simulink model "dds_cwg_32k_nb_half"  (R2018a)
settings: Solver=VariableStepDiscrete  StartTime=0.0  StopTime=(2^16)*20  RelTol=1e-3
undefined symbols (not defined in the file or in its folder): fft_stages, pfb_coeff_gen_calc
libraries: xbsIndex_r4 x11238, casper_library_misc x13, casper_library_delays x2, xps_library x1
(part 2 of 69)

== system dds_cwg_32k_nb_half/DDC ==
  note: DDS 18.17
  note: Mixer
  note: Filter
  note: Sync and DV will be inline here
  note: Sync and DV will be inline here
  sync : Inport
  dvalid : Inport  Port=2
  pol0_data : Inport  Port=3
  osc0 : Inport  Port=4
  pol1_data : Inport  Port=5
  osc1 : Inport  Port=6
  Assert1 : xbsIndex_r4/Assert  assert_type=on  type_source=Explicitly  gui_display_data_type=Boolean  arith_type=Boolean  n_bits=16  bin_pt=14  preci_type=Single  exp_width=8  frac_width=24  assert_rate=off  rate_source=Explicitly  period=1  output_port=on  block_type=assert
  Concat : xbsIndex_r4/Concat  num_inputs=2  dbl_ovrd=off  block_type=concat
  Concat1 : xbsIndex_r4/Concat  num_inputs=2  dbl_ovrd=off  block_type=concat
  Constant : xbsIndex_r4/Constant  const=0  gui_display_data_type=Fixed-point  arith_type=Unsigned  n_bits=1  bin_pt=0  preci_type=Single  exp_width=8  frac_width=24  explicit_period=on  period=1  equ=P=C  opselect=C  inp2=PCIN>>17  opr=+  inp1=P  carry=CIN  dbl_ovrd=off  block_type=constant
  Counter1 : xbsIndex_r4/Counter  Commented=on  cnt_type=Free Running  cnt_to=Inf  operation=Up  start_count=0  cnt_by_val=1  arith_type=Unsigned  n_bits=8  bin_pt=0  load_pin=off  rst=on  en=on  explicit_period=on  period=1  use_behavioral_HDL=off  implementation=DSP48  dbl_ovrd=off  block_type=counter
      settings: block_version=11.4
  Counter3 : xbsIndex_r4/Counter  Commented=on  cnt_type=Free Running  cnt_to=Inf  operation=Up  start_count=0  cnt_by_val=1  arith_type=Unsigned  n_bits=8  bin_pt=0  load_pin=off  rst=on  en=on  explicit_period=on  period=1  use_behavioral_HDL=off  implementation=DSP48  dbl_ovrd=off  block_type=counter
      settings: block_version=11.4
  Delay{1,9..13,15} (7 alike) : xbsIndex_r4/Delay  rst=off  infoeditControl=Selection of Reset will increase slice count due to use of real FFs and instead of SRLs  en=off  latency=1  reg_retiming=off  dbl_ovrd=off  block_type=delay
      settings: infoedit=Hardware notes: A delay line is a chain, each link of which is an SRL16 or SRL32 followed by a flip-flop.
  Delay14 : xbsIndex_r4/Delay  rst=off  infoeditControl=Selection of Reset will increase slice count due to use of real FFs and instead of SRLs  en=on  latency=2  reg_retiming=off  dbl_ovrd=off  block_type=delay
  Delay3 : xbsIndex_r4/Delay  rst=off  infoeditControl=Selection of Reset will increase slice count due to use of real FFs and instead of SRLs  en=on  latency=3  reg_retiming=off  dbl_ovrd=off  block_type=delay
  Delay4 : xbsIndex_r4/Delay  rst=off  infoeditControl=Selection of Reset will increase slice count due to use of real FFs and instead of SRLs  en=on  latency=1  reg_retiming=off  dbl_ovrd=off  block_type=delay
      settings: infoedit=Hardware notes: A delay line is a chain, each link of which is an SRL16 or SRL32 followed by a flip-flop.
  Delay5 : xbsIndex_r4/Delay  rst=off  infoeditControl=Selection of Reset will increase slice count due to use of real FFs and instead of SRLs  en=on  latency=3  reg_retiming=off  dbl_ovrd=off  block_type=delay
  Delay7 : xbsIndex_r4/Delay  rst=off  infoeditControl=Selection of Reset will increase slice count due to use of real FFs and instead of SRLs  en=on  latency=1  reg_retiming=off  dbl_ovrd=off  block_type=delay
      settings: infoedit=Hardware notes: A delay line is a chain, each link of which is an SRL16 or SRL32 followed by a flip-flop.
  Delay8 : xbsIndex_r4/Delay  rst=off  infoeditControl=Selection of Reset will increase slice count due to use of real FFs and instead of SRLs  en=on  latency=2  reg_retiming=off  dbl_ovrd=off  block_type=delay
  From16 : From  Commented=on  GotoTag=mix_80_0  TagVisibility=global
  From20 : From  Commented=on  GotoTag=cnt_rst  TagVisibility=global
      settings: CloseFcn=tagdialog Close
  From28 : From  Commented=on  GotoTag=cnt_rst  TagVisibility=global
      settings: CloseFcn=tagdialog Close
  From33 : From  Commented=on  GotoTag=dec_sync  TagVisibility=global
  From34 : From  Commented=on  GotoTag=ddc_sync
  Gateway Out{1..2,4,22..23} (5 alike) : xbsIndex_r4/Gateway Out  inherit_from_input=off  hdl_port=on  rows=1  columns=1  UseAsDAC=off  DACChannel='1'  interface=None  automatic_assignment=on  address_offset=hex2dec('00')  intf_name=''  intf_description=''  timing_constraint=None  locs_specified=off  LOCs={}  io_standard={}  block_type=gatewayout
  Gateway Out{10,12..21,24..28} (16 alike) : xbsIndex_r4/Gateway Out  Commented=on  inherit_from_input=off  hdl_port=on  rows=1  columns=1  UseAsDAC=off  DACChannel='1'  interface=None  automatic_assignment=on  address_offset=hex2dec('00')  intf_name=''  intf_description=''  timing_constraint=None  locs_specified=off  LOCs={}  io_standard={}  block_type=gatewayout
  Inverter1 : xbsIndex_r4/Inverter  en=off  latency=0  dbl_ovrd=off  block_type=inv
  Logical : xbsIndex_r4/Logical  Commented=on  logical_function=OR  inputs=2  en=off  latency=0  precision=Full  arith_type=Unsigned  n_bits=16  bin_pt=0  align_bp=on  dbl_ovrd=off  block_type=logical
  Logical3 : xbsIndex_r4/Logical  logical_function=AND  inputs=2  en=off  latency=1  precision=Full  arith_type=Unsigned  n_bits=16  bin_pt=0  align_bp=on  dbl_ovrd=off  block_type=logical
  Logical4 : xbsIndex_r4/Logical  logical_function=AND  inputs=2  en=off  latency=0  precision=Full  arith_type=Unsigned  n_bits=16  bin_pt=0  align_bp=on  dbl_ovrd=off  block_type=logical
  Register4 : xbsIndex_r4/Register  init=0  rst=off  en=on  dbl_ovrd=off  block_type=register
  Register5 : xbsIndex_r4/Register  init=0  rst=on  en=on  dbl_ovrd=off  block_type=register
  Register6 : xbsIndex_r4/Register  init=0  rst=on  en=on  dbl_ovrd=off  block_type=register
  Register7 : xbsIndex_r4/Register  init=0  rst=off  en=on  dbl_ovrd=off  block_type=register
  Terminator : Terminator
  Terminator1 : Terminator
  To Workspace1 : ToWorkspace  VariableName=mult_sync  SaveFormat=Timeseries  SampleTime=-1
  To Workspace11 : ToWorkspace  Commented=on  VariableName=mix_r0  SaveFormat=Timeseries  SampleTime=-1
  To Workspace13 : ToWorkspace  Commented=on  VariableName=mix_i0  SaveFormat=Timeseries  SampleTime=-1
  To Workspace14 : ToWorkspace  Commented=on  VariableName=mix_r1  SaveFormat=Timeseries  SampleTime=-1
  To Workspace15 : ToWorkspace  Commented=on  VariableName=mix_r2  SaveFormat=Timeseries  SampleTime=-1
  To Workspace16 : ToWorkspace  Commented=on  VariableName=mix_r3  SaveFormat=Timeseries  SampleTime=-1
  To Workspace17 : ToWorkspace  Commented=on  VariableName=mix_r4  SaveFormat=Timeseries  SampleTime=-1
  To Workspace18 : ToWorkspace  Commented=on  VariableName=mix_r5  SaveFormat=Timeseries  SampleTime=-1
  To Workspace19 : ToWorkspace  Commented=on  VariableName=mix_r6  SaveFormat=Timeseries  SampleTime=-1
  To Workspace2 : ToWorkspace  VariableName=mult_dv  SaveFormat=Timeseries  SampleTime=-1
  To Workspace20 : ToWorkspace  Commented=on  VariableName=mix_r7  SaveFormat=Timeseries  SampleTime=-1
  To Workspace21 : ToWorkspace  Commented=on  VariableName=mix_i1  SaveFormat=Timeseries  SampleTime=-1
  To Workspace22 : ToWorkspace  VariableName=ddc_pol0_re1  SaveFormat=Timeseries  SampleTime=-1
  To Workspace23 : ToWorkspace  Commented=on  VariableName=mix_i2  SaveFormat=Timeseries  SampleTime=-1
  To Workspace24 : ToWorkspace  Commented=on  VariableName=mix_i3  SaveFormat=Timeseries  SampleTime=-1
  To Workspace25 : ToWorkspace  Commented=on  VariableName=mix_i4  SaveFormat=Timeseries  SampleTime=-1
  To Workspace26 : ToWorkspace  Commented=on  VariableName=mix_i5  SaveFormat=Timeseries  SampleTime=-1
  To Workspace27 : ToWorkspace  Commented=on  VariableName=mix_i6  SaveFormat=Timeseries  SampleTime=-1
  To Workspace28 : ToWorkspace  Commented=on  VariableName=mix_i7  SaveFormat=Timeseries  SampleTime=-1
  To Workspace4 : ToWorkspace  VariableName=ddc_half_sync  SaveFormat=Timeseries  SampleTime=-1
  To Workspace5 : ToWorkspace  VariableName=ddc_pol0_im1  SaveFormat=Timeseries  SampleTime=-1
  bus_expand : Subsystem  mask(bus_expand){mode=divisions of equal size, outputNum=2, outputWidth=1, outputBinaryPt=0, outputArithmeticType=2, show_format=off, outputToWorkspace=off, variablePrefix=out, outputToModelAsWell=on}
      mask prompts: outputNum "Number of outputs:"; outputWidth "Output width:"; outputBinaryPt "Output binary point position:"; outputArithmeticType "Output arithmetic type (ufix=0, fix=1, bool=2):"; show_format "Print format string?"; outputToWorkspace "Output to workspace?"; variablePrefix "Variable name prefix:"; outputToModelAsWell "Output to model as well?"
      mask help:
      | Expands a 'bus' made using a bus_create or Xilinx
      | concat block.
      | The input will be divided into the specified number
      | of outputs with the specified arithmetic types.
      | Divisions are made from most significant bit.
      mask init: same as dds_cwg_32k_nb_half/bus_expand1
      settings: AttributesFormatString=2 outputs
      mask TypeOptions mode: divisions of equal size | divisions of arbitrary size
      mask Callback mode: bus_expand_callback();
      mask Callback outputWidth: bus_expand_callback();
      mask Callback outputToWorkspace: bus_expand_callback();
  bus_expand1 : Subsystem  mask(bus_expand){mode=divisions of equal size, outputNum=16, outputWidth=18, outputBinaryPt=17, outputArithmeticType=1, show_format=off, outputToWorkspace=off, variablePrefix=Sin, outputToModelAsWell=off}
      mask prompts: outputNum "Number of outputs:"; outputWidth "Output width:"; outputBinaryPt "Output binary point position:"; outputArithmeticType "Output arithmetic type (ufix=0, fix=1, bool=2):"; show_format "Print format string?"; outputToWorkspace "Output to workspace?"; variablePrefix "Variable name prefix:"; outputToModelAsWell "Output to model as well?"
      mask help:
      | Expands a 'bus' made using a bus_create or Xilinx
      | concat block.
      | The input will be divided into the specified number
      | of outputs with the specified arithmetic types.
      | Divisions are made from most significant bit.
      mask init: same as dds_cwg_32k_nb_half/bus_expand1
      settings: AttributesFormatString=16 outputs
      mask TypeOptions mode: divisions of equal size | divisions of arbitrary size
      mask Callback mode: bus_expand_callback();
      mask Callback outputWidth: bus_expand_callback();
      mask Callback outputToWorkspace: bus_expand_callback();
  bus_expand10 : Subsystem  mask(bus_expand){mode=divisions of equal size, outputNum=16, outputWidth=18, outputBinaryPt=17, outputArithmeticType=1, show_format=off, outputToWorkspace=off, variablePrefix=Sin, outputToModelAsWell=off}
      mask prompts: outputNum "Number of outputs:"; outputWidth "Output width:"; outputBinaryPt "Output binary point position:"; outputArithmeticType "Output arithmetic type (ufix=0, fix=1, bool=2):"; show_format "Print format string?"; outputToWorkspace "Output to workspace?"; variablePrefix "Variable name prefix:"; outputToModelAsWell "Output to model as well?"
      mask help:
      | Expands a 'bus' made using a bus_create or Xilinx
      | concat block.
      | The input will be divided into the specified number
      | of outputs with the specified arithmetic types.
      | Divisions are made from most significant bit.
      mask init: same as dds_cwg_32k_nb_half/bus_expand1
      settings: AttributesFormatString=16 outputs
      mask TypeOptions mode: divisions of equal size | divisions of arbitrary size
      mask Callback mode: bus_expand_callback();
      mask Callback outputWidth: bus_expand_callback();
      mask Callback outputToWorkspace: bus_expand_callback();
  bus_expand2 : Subsystem  mask(bus_expand){mode=divisions of equal size, outputNum=16, outputWidth=18, outputBinaryPt=17, outputArithmeticType=1, show_format=off, outputToWorkspace=off, variablePrefix=Sin, outputToModelAsWell=off}
      mask prompts: outputNum "Number of outputs:"; outputWidth "Output width:"; outputBinaryPt "Output binary point position:"; outputArithmeticType "Output arithmetic type (ufix=0, fix=1, bool=2):"; show_format "Print format string?"; outputToWorkspace "Output to workspace?"; variablePrefix "Variable name prefix:"; outputToModelAsWell "Output to model as well?"
      mask help:
      | Expands a 'bus' made using a bus_create or Xilinx
      | concat block.
      | The input will be divided into the specified number
      | of outputs with the specified arithmetic types.
      | Divisions are made from most significant bit.
      mask init: same as dds_cwg_32k_nb_half/bus_expand1
      settings: AttributesFormatString=16 outputs
      mask TypeOptions mode: divisions of equal size | divisions of arbitrary size
      mask Callback mode: bus_expand_callback();
      mask Callback outputWidth: bus_expand_callback();
      mask Callback outputToWorkspace: bus_expand_callback();
  bus_expand3 : Subsystem  mask(bus_expand){mode=divisions of equal size, outputNum=16, outputWidth=18, outputBinaryPt=17, outputArithmeticType=1, show_format=off, outputToWorkspace=off, variablePrefix=Sin, outputToModelAsWell=off}
      mask prompts: outputNum "Number of outputs:"; outputWidth "Output width:"; outputBinaryPt "Output binary point position:"; outputArithmeticType "Output arithmetic type (ufix=0, fix=1, bool=2):"; show_format "Print format string?"; outputToWorkspace "Output to workspace?"; variablePrefix "Variable name prefix:"; outputToModelAsWell "Output to model as well?"
      mask help:
      | Expands a 'bus' made using a bus_create or Xilinx
      | concat block.
      | The input will be divided into the specified number
      | of outputs with the specified arithmetic types.
      | Divisions are made from most significant bit.
      mask init: same as dds_cwg_32k_nb_half/bus_expand1
      settings: AttributesFormatString=16 outputs
      mask TypeOptions mode: divisions of equal size | divisions of arbitrary size
      mask Callback mode: bus_expand_callback();
      mask Callback outputWidth: bus_expand_callback();
      mask Callback outputToWorkspace: bus_expand_callback();
  bus_expand4 : Subsystem  mask(bus_expand){mode=divisions of equal size, outputNum=16, outputWidth=18, outputBinaryPt=17, outputArithmeticType=1, show_format=off, outputToWorkspace=off, variablePrefix=Sin, outputToModelAsWell=off}
      mask prompts: outputNum "Number of outputs:"; outputWidth "Output width:"; outputBinaryPt "Output binary point position:"; outputArithmeticType "Output arithmetic type (ufix=0, fix=1, bool=2):"; show_format "Print format string?"; outputToWorkspace "Output to workspace?"; variablePrefix "Variable name prefix:"; outputToModelAsWell "Output to model as well?"
      mask help:
      | Expands a 'bus' made using a bus_create or Xilinx
      | concat block.
      | The input will be divided into the specified number
      | of outputs with the specified arithmetic types.
      | Divisions are made from most significant bit.
      mask init: same as dds_cwg_32k_nb_half/bus_expand1
      settings: AttributesFormatString=16 outputs
      mask TypeOptions mode: divisions of equal size | divisions of arbitrary size
      mask Callback mode: bus_expand_callback();
      mask Callback outputWidth: bus_expand_callback();
      mask Callback outputToWorkspace: bus_expand_callback();
  bus_expand5 : Subsystem  mask(bus_expand){mode=divisions of equal size, outputNum=16, outputWidth=18, outputBinaryPt=17, outputArithmeticType=1, show_format=off, outputToWorkspace=off, variablePrefix=Sin, outputToModelAsWell=off}
      mask prompts: outputNum "Number of outputs:"; outputWidth "Output width:"; outputBinaryPt "Output binary point position:"; outputArithmeticType "Output arithmetic type (ufix=0, fix=1, bool=2):"; show_format "Print format string?"; outputToWorkspace "Output to workspace?"; variablePrefix "Variable name prefix:"; outputToModelAsWell "Output to model as well?"
      mask help:
      | Expands a 'bus' made using a bus_create or Xilinx
      | concat block.
      | The input will be divided into the specified number
      | of outputs with the specified arithmetic types.
      | Divisions are made from most significant bit.
      mask init: same as dds_cwg_32k_nb_half/bus_expand1
      settings: AttributesFormatString=16 outputs
      mask TypeOptions mode: divisions of equal size | divisions of arbitrary size
      mask Callback mode: bus_expand_callback();
      mask Callback outputWidth: bus_expand_callback();
      mask Callback outputToWorkspace: bus_expand_callback();
  bus_expand6 : Subsystem  mask(bus_expand){mode=divisions of equal size, outputNum=16, outputWidth=18, outputBinaryPt=17, outputArithmeticType=1, show_format=off, outputToWorkspace=off, variablePrefix=Sin, outputToModelAsWell=off}
      mask prompts: outputNum "Number of outputs:"; outputWidth "Output width:"; outputBinaryPt "Output binary point position:"; outputArithmeticType "Output arithmetic type (ufix=0, fix=1, bool=2):"; show_format "Print format string?"; outputToWorkspace "Output to workspace?"; variablePrefix "Variable name prefix:"; outputToModelAsWell "Output to model as well?"
      mask help:
      | Expands a 'bus' made using a bus_create or Xilinx
      | concat block.
      | The input will be divided into the specified number
      | of outputs with the specified arithmetic types.
      | Divisions are made from most significant bit.
      mask init: same as dds_cwg_32k_nb_half/bus_expand1
      settings: AttributesFormatString=16 outputs
      mask TypeOptions mode: divisions of equal size | divisions of arbitrary size
      mask Callback mode: bus_expand_callback();
      mask Callback outputWidth: bus_expand_callback();
      mask Callback outputToWorkspace: bus_expand_callback();
  bus_expand7 : Subsystem  AncestorBlock=casper_library_flow_control/bus_expand  mask(bus_expand){mode=divisions of equal size, outputNum=2, outputWidth=18, outputBinaryPt=17, outputArithmeticType=1, show_format=off, outputToWorkspace=off, variablePrefix=out, outputToModelAsWell=on}
      mask prompts: outputNum "Number of outputs:"; outputWidth "Output width:"; outputBinaryPt "Output binary point position:"; outputArithmeticType "Output arithmetic type (ufix=0, fix=1, bool=2):"; show_format "Print format string?"; outputToWorkspace "Output to workspace?"; variablePrefix "Variable name prefix:"; outputToModelAsWell "Output to model as well?"
      mask help:
      | Expands a 'bus' made using a bus_create or Xilinx
      | concat block.
      | The input will be divided into the specified number
      | of outputs with the specified arithmetic types.
      | Divisions are made from most significant bit.
      mask init: same as dds_cwg_32k_nb_half/bus_expand1
      settings: AttributesFormatString=2 outputs
      mask TypeOptions mode: divisions of equal size | divisions of arbitrary size
      mask Callback mode: bus_expand_callback();
      mask Callback outputWidth: bus_expand_callback();
      mask Callback outputToWorkspace: bus_expand_callback();
  bus_expand8 : Subsystem  Commented=on  mask(bus_expand){mode=divisions of equal size, outputNum=16, outputWidth=18, outputBinaryPt=17, outputArithmeticType=1, show_format=off, outputToWorkspace=off, variablePrefix=Sin, outputToModelAsWell=off}
      mask prompts: outputNum "Number of outputs:"; outputWidth "Output width:"; outputBinaryPt "Output binary point position:"; outputArithmeticType "Output arithmetic type (ufix=0, fix=1, bool=2):"; show_format "Print format string?"; outputToWorkspace "Output to workspace?"; variablePrefix "Variable name prefix:"; outputToModelAsWell "Output to model as well?"
      mask help:
      | Expands a 'bus' made using a bus_create or Xilinx
      | concat block.
      | The input will be divided into the specified number
      | of outputs with the specified arithmetic types.
      | Divisions are made from most significant bit.
      mask init: same as dds_cwg_32k_nb_half/bus_expand1
      settings: AttributesFormatString=16 outputs
      mask TypeOptions mode: divisions of equal size | divisions of arbitrary size
      mask Callback mode: bus_expand_callback();
      mask Callback outputWidth: bus_expand_callback();
      mask Callback outputToWorkspace: bus_expand_callback();
  bus_expand9 : Subsystem  mask(bus_expand){mode=divisions of equal size, outputNum=16, outputWidth=18, outputBinaryPt=17, outputArithmeticType=1, show_format=off, outputToWorkspace=off, variablePrefix=Sin, outputToModelAsWell=off}
      mask prompts: outputNum "Number of outputs:"; outputWidth "Output width:"; outputBinaryPt "Output binary point position:"; outputArithmeticType "Output arithmetic type (ufix=0, fix=1, bool=2):"; show_format "Print format string?"; outputToWorkspace "Output to workspace?"; variablePrefix "Variable name prefix:"; outputToModelAsWell "Output to model as well?"
      mask help:
      | Expands a 'bus' made using a bus_create or Xilinx
      | concat block.
      | The input will be divided into the specified number
      | of outputs with the specified arithmetic types.
      | Divisions are made from most significant bit.
      mask init: same as dds_cwg_32k_nb_half/bus_expand1
      settings: AttributesFormatString=16 outputs
      mask TypeOptions mode: divisions of equal size | divisions of arbitrary size
      mask Callback mode: bus_expand_callback();
      mask Callback outputWidth: bus_expand_callback();
      mask Callback outputToWorkspace: bus_expand_callback();
  bus_mult : Subsystem  mask(bus_mult){n_bits_a=[10,10,10,10,10,10,10,10], bin_pt_a=9, type_a=1, cmplx_a=on, n_bits_b=[18,18,18,18,18,18,18,18], bin_pt_b=17, type_b=1, cmplx_b=on, misc=on, floating_point=off, float_type=single, input_vec_a=1, input_vec_b=1, frac_width=19, exp_width=6, n_bits_out=18, bin_pt_out=17, type_out=1, quantization=1, overflow=0, mult_latency=7, add_latency=7, conv_latency=7, max_fanout=1, fan_latency=3, multiplier_implementation=embedded multiplier core, pipeline_cmult_en=off, pipeline_latency=0}
      mask prompts: n_bits_a "a input bit widths"; bin_pt_a "a input binary points"; type_a "a input type (Unsigned=0, Signed=1)"; cmplx_a "a input complex"; n_bits_b "b input bit widths"; bin_pt_b "b input binary points"; type_b "b input type (Unsigned=0, Signed=1)"; cmplx_b "b input complex"; misc "misc support"; floating_point "floating point"; float_type "float type"; input_vec_a "a input vector in bus"; input_vec_b "b input vector in bus"; frac_width "fraction width"; exp_width "exponent width"; n_bits_out "output bit widths"; bin_pt_out "output binary points"; type_out "output type (Unsigned=0, Signed=1)"; quantization "quantization strategy (Truncate=0, Round  (unbiased: +/- Inf)=1)"; overflow "overflow strategy (Wrap=0, Saturate=1, Flag as error=2)"; mult_latency "multiplier latency"; add_latency "adder latency"; conv_latency "convert latency"; max_fanout "limit fanout to ?"; fan_latency "fanout register latency"; multiplier_implementation "multiplier implementation"; pipeline_cmult_en "pipeline complex mult"; pipeline_latency "pipeline latency"
      mask help: Multiply components of two busses
      mask init:
      | bus_mult_init(gcb, ...
      |     'n_bits_a', n_bits_a, ...
      |     'bin_pt_a', bin_pt_a, ...
      |     'type_a', type_a, ...
      |     'cmplx_a', cmplx_a, ...
      |     'n_bits_b', n_bits_b, ...
      |     'bin_pt_b', bin_pt_b, ...
      |     'type_b', type_b, ...
      |     'cmplx_b', cmplx_b, ...
      |     'n_bits_out', n_bits_out, ...
      |     'bin_pt_out', bin_pt_out, ...
      |     'type_out', type_out, ...
      |     'floating_point', floating_point, ...
      |     'float_type', float_type, ...
      |     'exp_width', exp_width, ...
      |     'input_vec_a', input_vec_a, ...
      |     'input_vec_b', input_vec_b, ...
      |     'frac_width', frac_width, ...         
      |     'quantization', quantization, ...
      |     'overflow', overflow, ...
      |     'mult_latency', mult_latency, ...
      |     'add_latency', add_latency, ...
      |     'conv_latency', conv_latency, ...
      |     'max_fanout', max_fanout, ...
      |     'pipeline_cmult_en', pipeline_cmult_en, ...
      |     'pipeline_latency', pipeline_latency, ...
      |     'fan_latency', fan_latency, ...
      |     'multiplier_implementation', multiplier_implementation, ...
      |     'misc', misc);
      mask Callback floating_point:
      | onoff = get_param(gcb, 'floating_point');
      | if strcmp(onoff,'on')
      |     enable_fixpt = 'off'
      |     set_param_state(gcb, 'float_type', 'on')
      | 
      |     set_param_state(gcb, 'input_vec_a', 'on')
      |     set_param_state(gcb, 'input_vec_b', 'on')
      | 
      |     f_type = get_param(gcb, 'float_type')
      |     if strcmp(f_type,'custom')
      |         set_param_state(gcb, 'exp_width', 'on')
      |         set_param_state(gcb, 'frac_width', 'on')
      |     else
      |         set_param_state(gcb, 'exp_width', 'off')
      |         set_param_state(gcb, 'frac_width', 'off')
      |     end
      | 
      | else
      |     enable_fixpt = 'on'
      |     set_param_state(gcb, 'float_type', 'off')
      |     set_param_state(gcb, 'exp_width', 'off')
      |     set_param_state(gcb, 'frac_width', 'off')
      |     set_param_state(gcb, 'input_vec_a', 'off')
      |     set_param_state(gcb, 'input_vec_b', 'off')
      | end
      | 
      | set_param_state(gcb, 'n_bits_a', enable_fixpt)
      | set_param_state(gcb, 'bin_pt_a', enable_fixpt)
      | set_param_state(gcb, 'type_a', enable_fixpt)
      | set_param_state(gcb, 'n_bits_b', enable_fixpt)
      | set_param_state(gcb, 'bin_pt_b', enable_fixpt)
      | set_param_state(gcb, 'type_b', enable_fixpt)
      | 
      | set_param_state(gcb, 'n_bits_out', enable_fixpt)
      | set_param_state(gcb, 'bin_pt_out', enable_fixpt)
      | set_param_state(gcb, 'type_out', enable_fixpt)
      | set_param_state(gcb, 'quantization', enable_fixpt)
      | set_param_state(gcb, 'overflow', enable_fixpt)
      mask TypeOptions float_type: single | custom
      mask Callback float_type:
      | f_type = get_param(gcb, 'float_type')
      | if strcmp(f_type,'custom')
      |     set_param_state(gcb, 'exp_width', 'on')
      |     set_param_state(gcb, 'frac_width', 'on')
      | else
      |     set_param_state(gcb, 'exp_width', 'off')
      |     set_param_state(gcb, 'frac_width', 'off')
      | end
      mask TypeOptions multiplier_implementation: behavioral HDL | standard core | embedded multiplier core
      mask Callback pipeline_cmult_en:
      | pipeline_en = get_param(gcb, 'pipeline_cmult_en');
      | if strcmp(pipeline_en,'on')
      | 
      |     set_param_state(gcb, 'pipeline_latency', 'on')
      | else
      |     set_param_state(gcb, 'pipeline_latency', 'off')
      | end
  bus_mult1 : Subsystem  mask(bus_mult){n_bits_a=[10,10,10,10,10,10,10,10], bin_pt_a=9, type_a=1, cmplx_a=on, n_bits_b=[18,18,18,18,18,18,18,18], bin_pt_b=17, type_b=1, cmplx_b=on, misc=off, floating_point=off, float_type=single, input_vec_a=1, input_vec_b=1, frac_width=19, exp_width=6, n_bits_out=18, bin_pt_out=17, type_out=1, quantization=1, overflow=0, mult_latency=7, add_latency=7, conv_latency=7, max_fanout=1, fan_latency=3, multiplier_implementation=embedded multiplier core, pipeline_cmult_en=off, pipeline_latency=0}
      mask prompts: n_bits_a "a input bit widths"; bin_pt_a "a input binary points"; type_a "a input type (Unsigned=0, Signed=1)"; cmplx_a "a input complex"; n_bits_b "b input bit widths"; bin_pt_b "b input binary points"; type_b "b input type (Unsigned=0, Signed=1)"; cmplx_b "b input complex"; misc "misc support"; floating_point "floating point"; float_type "float type"; input_vec_a "a input vector in bus"; input_vec_b "b input vector in bus"; frac_width "fraction width"; exp_width "exponent width"; n_bits_out "output bit widths"; bin_pt_out "output binary points"; type_out "output type (Unsigned=0, Signed=1)"; quantization "quantization strategy (Truncate=0, Round  (unbiased: +/- Inf)=1)"; overflow "overflow strategy (Wrap=0, Saturate=1, Flag as error=2)"; mult_latency "multiplier latency"; add_latency "adder latency"; conv_latency "convert latency"; max_fanout "limit fanout to ?"; fan_latency "fanout register latency"; multiplier_implementation "multiplier implementation"; pipeline_cmult_en "pipeline complex mult"; pipeline_latency "pipeline latency"
      mask help: Multiply components of two busses
      mask init: same as dds_cwg_32k_nb_half/DDC/bus_mult
      mask Callback floating_point:
      | onoff = get_param(gcb, 'floating_point');
      | if strcmp(onoff,'on')
      |     enable_fixpt = 'off'
      |     set_param_state(gcb, 'float_type', 'on')
      | 
      |     set_param_state(gcb, 'input_vec_a', 'on')
      |     set_param_state(gcb, 'input_vec_b', 'on')
      | 
      |     f_type = get_param(gcb, 'float_type')
      |     if strcmp(f_type,'custom')
      |         set_param_state(gcb, 'exp_width', 'on')
      |         set_param_state(gcb, 'frac_width', 'on')
      |     else
      |         set_param_state(gcb, 'exp_width', 'off')
      |         set_param_state(gcb, 'frac_width', 'off')
      |     end
      | 
      | else
      |     enable_fixpt = 'on'
      |     set_param_state(gcb, 'float_type', 'off')
      |     set_param_state(gcb, 'exp_width', 'off')
      |     set_param_state(gcb, 'frac_width', 'off')
      |     set_param_state(gcb, 'input_vec_a', 'off')
      |     set_param_state(gcb, 'input_vec_b', 'off')
      | end
      | 
      | set_param_state(gcb, 'n_bits_a', enable_fixpt)
      | set_param_state(gcb, 'bin_pt_a', enable_fixpt)
      | set_param_state(gcb, 'type_a', enable_fixpt)
      | set_param_state(gcb, 'n_bits_b', enable_fixpt)
      | set_param_state(gcb, 'bin_pt_b', enable_fixpt)
      | set_param_state(gcb, 'type_b', enable_fixpt)
      | 
      | set_param_state(gcb, 'n_bits_out', enable_fixpt)
      | set_param_state(gcb, 'bin_pt_out', enable_fixpt)
      | set_param_state(gcb, 'type_out', enable_fixpt)
      | set_param_state(gcb, 'quantization', enable_fixpt)
      | set_param_state(gcb, 'overflow', enable_fixpt)
      mask TypeOptions float_type: single | custom
      mask Callback float_type:
      | f_type = get_param(gcb, 'float_type')
      | if strcmp(f_type,'custom')
      |     set_param_state(gcb, 'exp_width', 'on')
      |     set_param_state(gcb, 'frac_width', 'on')
      | else
      |     set_param_state(gcb, 'exp_width', 'off')
      |     set_param_state(gcb, 'frac_width', 'off')
      | end
      mask TypeOptions multiplier_implementation: behavioral HDL | standard core | embedded multiplier core
      mask Callback pipeline_cmult_en:
      | pipeline_en = get_param(gcb, 'pipeline_cmult_en');
      | if strcmp(pipeline_en,'on')
      | 
      |     set_param_state(gcb, 'pipeline_latency', 'on')
      | else
      |     set_param_state(gcb, 'pipeline_latency', 'off')
      | end
  convert_of : Subsystem  Commented=on  AncestorBlock=casper_library_misc/convert_of  mask(convert_of){bit_width_i=44, binary_point_i=34, bit_width_o=18, binary_point_o=17, latency=2, overflow=Saturate, quantization=Round  (unbiased: +/- Inf)}
      mask prompts: bit_width_i "Bit Width In"; binary_point_i "Binary Point In"; bit_width_o "Bit Width Out"; binary_point_o "Binary Point Out"; overflow "Overflow Behaviour"; quantization "Quantization Behaviour"
      mask help:
      | Converts from one 2's complement bit-width
      | and/or binary point position to another.
      | Includes underflow/overflow indicator.
      mask init:
      | convert_of_init(gcb, ...
      |     'bit_width_i', bit_width_i, ...
      |     'binary_point_i', binary_point_i, ...
      |     'bit_width_o', bit_width_o, ...
      |     'binary_point_o', binary_point_o, ...
      |     'latency', latency, ...
      |     'overflow', overflow, ...
      |     'quantization', quantization);
      settings: AttributesFormatString=[44,34]->[18,17]
      mask TypeOptions overflow: Wrap | Saturate | Error
      mask TypeOptions quantization: Truncate | Round  (unbiased: +/- Inf) | Round  (unbiased: even values)
  convert_of1 : Subsystem  Commented=on  AncestorBlock=casper_library_misc/convert_of  mask(convert_of){bit_width_i=44, binary_point_i=34, bit_width_o=18, binary_point_o=17, latency=2, overflow=Saturate, quantization=Round  (unbiased: +/- Inf)}
      mask prompts: bit_width_i "Bit Width In"; binary_point_i "Binary Point In"; bit_width_o "Bit Width Out"; binary_point_o "Binary Point Out"; overflow "Overflow Behaviour"; quantization "Quantization Behaviour"
      mask help:
      | Converts from one 2's complement bit-width
      | and/or binary point position to another.
      | Includes underflow/overflow indicator.
      mask init: same as dds_cwg_32k_nb_half/DDC/convert_of
      settings: AttributesFormatString=[44,34]->[18,17]
      mask TypeOptions overflow: Wrap | Saturate | Error
      mask TypeOptions quantization: Truncate | Round  (unbiased: +/- Inf) | Round  (unbiased: even values)
  ddc_in_sync_cnt : Subsystem  Tag=xps:sw_reg  Commented=on  AncestorBlock=xps_library/Memory/software_register  mask(swreg){io_dir=To Processor, io_delay=0, init_val=0, sample_period=1, names=reg, bitwidths=8, bin_pts=0, arith_types=0, sim_port=off, show_format=on}
      mask prompts: io_dir "I/O direction"; io_delay "I/O delay"; init_val "Initial Value"; sample_period "Sample period"; names "Bitfield names [msb...lsb]"; bitwidths "Bitfield widths"; bin_pts "Bitfield binary pts"; arith_types "Bitfield types, ufix=0, fix=1, bool=2"; sim_port "Provide sim input/output?"; show_format "Print format string?"
      mask help: A 32-bit software-accessible register. Can be divided into bitfields of varying widths and types using the fields in the block mask.
      mask init:
      | swreg_init(gcb)
      settings: AttributesFormatString=1output:uf8.0 = 8 bits
      mask TypeOptions io_dir: To Processor | From Processor
      mask Callback io_dir:
      | mask_enables = get_param(gcb, 'MaskEnables');
      | mask_names = get_param(gcb, 'MaskNames');
      | if strcmp(get_param(gcb, 'io_dir'), 'To Processor'),
      |     mask_enables{ismember(mask_names, 'sample_period')} = 'off';
      | else
      |     mask_enables{ismember(mask_names, 'sample_period')} = 'on';
      | end
      | set_param(gcb, 'MaskEnables', mask_enables);
      mask DialogControl ParameterTabVar0 Prompt: Setup
  ddc_out_sync_cnt : Subsystem  Tag=xps:sw_reg  Commented=on  AncestorBlock=xps_library/Memory/software_register  mask(swreg){io_dir=To Processor, io_delay=0, init_val=0, sample_period=1, names=reg, bitwidths=8, bin_pts=0, arith_types=0, sim_port=off, show_format=on}
      mask prompts: io_dir "I/O direction"; io_delay "I/O delay"; init_val "Initial Value"; sample_period "Sample period"; names "Bitfield names [msb...lsb]"; bitwidths "Bitfield widths"; bin_pts "Bitfield binary pts"; arith_types "Bitfield types, ufix=0, fix=1, bool=2"; sim_port "Provide sim input/output?"; show_format "Print format string?"
      mask help: A 32-bit software-accessible register. Can be divided into bitfields of varying widths and types using the fields in the block mask.
      mask init:
      | swreg_init(gcb)
      settings: AttributesFormatString=1output:uf8.0 = 8 bits
      mask TypeOptions io_dir: To Processor | From Processor
      mask Callback io_dir:
      | mask_enables = get_param(gcb, 'MaskEnables');
      | mask_names = get_param(gcb, 'MaskNames');
      | if strcmp(get_param(gcb, 'io_dir'), 'To Processor'),
      |     mask_enables{ismember(mask_names, 'sample_period')} = 'off';
      | else
      |     mask_enables{ismember(mask_names, 'sample_period')} = 'on';
      | end
      | set_param(gcb, 'MaskEnables', mask_enables);
      mask DialogControl ParameterTabVar0 Prompt: Setup
  dec_fir_async1 : Subsystem  Tag=casper:dec_fir_async  AncestorBlock=casper_library_downconverter/dec_fir_async  mask(dec_fir_async){n_inputs=32, coeff=[-0.000339,-0.000234,-0.000312,-0.000402,-0.000507,-0.000626,-0.000760,-0.000909,-0.001071,-0.001247,-0.001436,-0.001634,-0.001841,-0.002054,-0.002269,-0.002483,-0.002692,-0.002892,-0.003077,-0.003243,-0.003383,-0.003491,-0.003562,-0.003589,-0.003566,-0.003487,-0.003345,-0.003135,-0.002850,-0.002487,-0.002040,-0.001506,-0.000881,-0.000163,0.000649,0.001555,0.002555,0.003646,0.004826,0.006089,0.007432,0.008847,0.010325,0.011860,0.013440,0.015055,0.016693,0.018341,0.019988,0.021620,0.023223,0.024783,0.026286,0.027720,0.029072,0.030327,0.031476,0.032507,0.033410,0.034177,0.034799,0.035272,0.035589,0.035749,0.035749,0.035589,0.035272,0.034799,0.034177,0.033410,0.032507,0.031476,0.030327,0.029072,0.027720,0.026286,0.024783,0.023223,0.021620,0.019988,0.018341,0.016693,0.015055,0.013440,0.011860,0.010325,0.008847,0.007432,0.006089,0.004826,0.003646,0.002555,0.001555,0.000649,-0.000163,-0.000881,-0.001506,-0.002040,-0.002487,-0.002850,-0.003135,-0.003345,-0.003487,-0.003566,-0.003589,-0.003562,-0.003491,-0.003383,-0.003243,-0.003077,-0.002892,-0.002692,-0.002483,-0.002269,-0.002054,-0.001841,-0.001634,-0.001436,-0.001247,-0.001071,-0.000909,-0.000760,-0.000626,-0.000507,-0.000402,-0.000312,-0.000234,-0.000339], output_width=18, output_bp=17, quantization=Round  (unbiased: +/- Inf), add_latency=7, mult_latency=7, conv_latency=7, coeff_bit_width=18, coeff_bin_pt=17, lshift=1, absorb_adders=on, adder_imp=DSP48, async=on, bus_input=off, input_width=0, input_bp=0, input_type=Signed}
      mask prompts: n_inputs "Number of Parallel Streams"; coeff "Coefficients"; output_width "Output bitwidth"; output_bp "Output binary point"; quantization "Quantization Behavior"; add_latency "Add Latency"; mult_latency "Mult Latency"; conv_latency "Convert latency"; coeff_bit_width "Coefficient bitwidth"; coeff_bin_pt "Coefficient binary point"; lshift "Post adder-tree shift"; absorb_adders "Absorb adders into DSP slices"; adder_imp "Adder implementation"; async "Asynchronous ops"; bus_input "Bus input"; input_width "Input bitwidth"; input_bp "Input binary point"; input_type "Input datatype"
      mask help: FIR filter which can handle multiple time samples in parallel and decimates down to 1 time sample. If coefficients are symmetric, will automatically fold before multiplying.
      mask init:
      | dec_fir_async_init(gcb);
      settings: AttributesFormatString=|
      | 128 taps
      | 18_17 r/i
      mask TypeOptions quantization: Truncate | Round  (unbiased: +/- Inf) | Round  (unbiased: Even Values)
      mask TypeOptions adder_imp: Behavioral | Fabric | DSP48
      mask Callback bus_input:
      | onoff = get_param(gcb, 'bus_input');
      | set_param_state(gcb, 'input_width', onoff)
      | set_param_state(gcb, 'input_bp', onoff)
      | set_param_state(gcb, 'input_type', onoff)
      mask TypeOptions input_type: Signed | Unsigned
  dec_fir_async2 : Subsystem  Tag=casper:dec_fir_async  AncestorBlock=casper_library_downconverter/dec_fir_async  mask(dec_fir_async){n_inputs=32, coeff=[-0.000339,-0.000234,-0.000312,-0.000402,-0.000507,-0.000626,-0.000760,-0.000909,-0.001071,-0.001247,-0.001436,-0.001634,-0.001841,-0.002054,-0.002269,-0.002483,-0.002692,-0.002892,-0.003077,-0.003243,-0.003383,-0.003491,-0.003562,-0.003589,-0.003566,-0.003487,-0.003345,-0.003135,-0.002850,-0.002487,-0.002040,-0.001506,-0.000881,-0.000163,0.000649,0.001555,0.002555,0.003646,0.004826,0.006089,0.007432,0.008847,0.010325,0.011860,0.013440,0.015055,0.016693,0.018341,0.019988,0.021620,0.023223,0.024783,0.026286,0.027720,0.029072,0.030327,0.031476,0.032507,0.033410,0.034177,0.034799,0.035272,0.035589,0.035749,0.035749,0.035589,0.035272,0.034799,0.034177,0.033410,0.032507,0.031476,0.030327,0.029072,0.027720,0.026286,0.024783,0.023223,0.021620,0.019988,0.018341,0.016693,0.015055,0.013440,0.011860,0.010325,0.008847,0.007432,0.006089,0.004826,0.003646,0.002555,0.001555,0.000649,-0.000163,-0.000881,-0.001506,-0.002040,-0.002487,-0.002850,-0.003135,-0.003345,-0.003487,-0.003566,-0.003589,-0.003562,-0.003491,-0.003383,-0.003243,-0.003077,-0.002892,-0.002692,-0.002483,-0.002269,-0.002054,-0.001841,-0.001634,-0.001436,-0.001247,-0.001071,-0.000909,-0.000760,-0.000626,-0.000507,-0.000402,-0.000312,-0.000234,-0.000339], output_width=18, output_bp=17, quantization=Round  (unbiased: +/- Inf), add_latency=7, mult_latency=7, conv_latency=7, coeff_bit_width=18, coeff_bin_pt=17, lshift=1, absorb_adders=on, adder_imp=DSP48, async=on, bus_input=off, input_width=0, input_bp=0, input_type=Signed}
      mask prompts: n_inputs "Number of Parallel Streams"; coeff "Coefficients"; output_width "Output bitwidth"; output_bp "Output binary point"; quantization "Quantization Behavior"; add_latency "Add Latency"; mult_latency "Mult Latency"; conv_latency "Convert latency"; coeff_bit_width "Coefficient bitwidth"; coeff_bin_pt "Coefficient binary point"; lshift "Post adder-tree shift"; absorb_adders "Absorb adders into DSP slices"; adder_imp "Adder implementation"; async "Asynchronous ops"; bus_input "Bus input"; input_width "Input bitwidth"; input_bp "Input binary point"; input_type "Input datatype"
      mask help: FIR filter which can handle multiple time samples in parallel and decimates down to 1 time sample. If coefficients are symmetric, will automatically fold before multiplying.
      mask init:
      | dec_fir_async_init(gcb);
      settings: AttributesFormatString=|
      | 128 taps
      | 18_17 r/i
      mask TypeOptions quantization: Truncate | Round  (unbiased: +/- Inf) | Round  (unbiased: Even Values)
      mask TypeOptions adder_imp: Behavioral | Fabric | DSP48
      mask Callback bus_input:
      | onoff = get_param(gcb, 'bus_input');
      | set_param_state(gcb, 'input_width', onoff)
      | set_param_state(gcb, 'input_bp', onoff)
      | set_param_state(gcb, 'input_type', onoff)
      mask TypeOptions input_type: Signed | Unsigned
  edge_detect2 : Subsystem  AncestorBlock=casper_library_misc/edge_detect  mask(edge_detect){edge=Rising, polarity=Active High, x_in=[0 0.08 0.08 0.16 0.16 0.24 0.24 0.32 0.32 0.4], y_in=[-1 -1  1  1  1  1  1  1  1  1], x_out=[0.6 0.68 0.68 0.76 0.76 0.84 0.84 0.92 0.92 1], y_out=[-1 -1  1  1 -1 -1 -1 -1 -1 -1]}
      mask prompts: edge "Edge Type"; polarity "Output Polarity"; x_in "Input X Positions"; y_in "Input Y Positions"; x_out "Output X Positions"; y_out "Output Y Positions"
      mask help: Output is active for one-cycle after each edge of the specified type (i.e. rising, falling or both).
      mask init: same as dds_cwg_32k_nb_half/edge_detect1
      settings: AttributesFormatString=|
      | rising edges
      | active high
      mask Help: Output is active for one-cycle after each edge of the specified type (i.e. rising, falling, or both).  Latency is zero.
      mask TypeOptions edge: Rising | Falling | Both
      mask TypeOptions polarity: Active High | Active Low
      mask Display:
      | plot(x_in_num,0.5+y_in_num*0.2);
      | plot(x_out_num,0.5+y_out_num*0.2);
  pipeline21 : Subsystem  Commented=on  AncestorBlock=casper_library_delays/pipeline  mask(pipeline){latency=2}
      mask help:
      | An explicitly laid-out delay line to avoid mapping to SRL16s
      | for use in pipelining to help achieve timing closure.
      mask init:
      | pipeline_init(gcb,'latency',latency);
      settings: AttributesFormatString=Latency = %<latency>
      mask Display:
      | port_label('input', 1, 'd');
      | port_label('output', 1, 'q');
      | disp(['Z^-', num2str(latency)]);
  pipeline22 : Subsystem  Commented=on  AncestorBlock=casper_library_delays/pipeline  mask(pipeline){latency=2}
      mask help:
      | An explicitly laid-out delay line to avoid mapping to SRL16s
      | for use in pipelining to help achieve timing closure.
      mask init:
      | pipeline_init(gcb,'latency',latency);
      settings: AttributesFormatString=Latency = %<latency>
      mask Display:
      | port_label('input', 1, 'd');
      | port_label('output', 1, 'q');
      | disp(['Z^-', num2str(latency)]);
  pipeline39 : Subsystem  Commented=on  AncestorBlock=casper_library_delays/pipeline  mask(pipeline){latency=2}
      mask help:
      | An explicitly laid-out delay line to avoid mapping to SRL16s
      | for use in pipelining to help achieve timing closure.
      mask init:
      | pipeline_init(gcb,'latency',latency);
      settings: AttributesFormatString=Latency = %<latency>
      mask Display:
      | port_label('input', 1, 'd');
      | port_label('output', 1, 'q');
      | disp(['Z^-', num2str(latency)]);
  pipeline40 : Subsystem  Commented=on  AncestorBlock=casper_library_delays/pipeline  mask(pipeline){latency=2}
      mask help:
      | An explicitly laid-out delay line to avoid mapping to SRL16s
      | for use in pipelining to help achieve timing closure.
      mask init:
      | pipeline_init(gcb,'latency',latency);
      settings: AttributesFormatString=Latency = %<latency>
      mask Display:
      | port_label('input', 1, 'd');
      | port_label('output', 1, 'q');
      | disp(['Z^-', num2str(latency)]);
  ri_to_c1 : casper_library_misc/ri_to_c  Commented=on
      settings: SourceProductName=CASPER DSP Blockset
  ddc_sync : Outport
  ddc_pol0 : Outport  Port=2
  ddc_pol1 : Outport  Port=3
  ddc_dv : Outport  Port=4
  ddc_of : Outport  Port=5
  tag scope: dec_d80_0=global, dec_d80_1=global, dec_dv=global, dec_sync=global, mix_80_0=global, mix_dvalid=global, mix_sync=global
  wires:
  Concat/1 -> bus_mult/3(misci)
  bus_mult/2(misco) -> bus_expand/1(bus_in)
  [ddc_sync] -> ddc_sync/1
  [ddc_pol0] -> ddc_pol0/1
  [ddc_pol1] -> ddc_pol1/1
  pol1_data/1 -> bus_mult1/1(a)
  osc1/1 -> bus_mult1/2(b)
  From20/1 -> pipeline22/1(d)
  Counter1/1 -> ddc_out_sync_cnt/1(out_reg)
  pipeline21/1(q) -> Counter1/2
  pipeline22/1(q) -> Counter1/1
  From34/1 -> pipeline21/1(d)
  [ddc_dvalid] -> ddc_dv/1
  From28/1 -> pipeline40/1(d)
  Counter3/1 -> ddc_in_sync_cnt/1(out_reg)
  pipeline39/1(q) -> Counter3/2
  pipeline40/1(q) -> Counter3/1
  From33/1 -> pipeline39/1(d)
  [ddc_of_pol0] -> Concat1/1
  [ddc_of_pol1] -> Concat1/2
  Concat1/1 -> ddc_of/1
  Constant/1 -> [ddc_of_pol1], [ddc_of_pol0]
  convert_of1/1(dout) -> ri_to_c1/2
  convert_of/1(dout) -> ri_to_c1/1
  convert_of/2(of) -> Logical/1
  convert_of1/2(of) -> Logical/2
  sync/1 -> Concat/1
  dvalid/1 -> Concat/2
  osc0/1 -> bus_mult/2(b)
  pol0_data/1 -> bus_mult/1(a)
  bus_expand/1(msb_out2) -> Gateway Out1/1, [mix_sync]
  Gateway Out1/1 -> To Workspace1/1
  Gateway Out2/1 -> To Workspace2/1
  bus_expand/2(lsb_out1) -> Gateway Out2/1, [mix_dvalid]
  bus_mult1/1(a*b) -> [mix_80_1]
  bus_mult/1(a*b) -> [mix_80_0]
  [dec_d80_0] -> Delay5/1, Delay8/1, Delay7/1, bus_expand4/1(bus_in)
  [dec_dv] -> dec_fir_async1/2(dv_in)
  [dec_sync] -> dec_fir_async1/1(sync_in)
  bus_expand1/1(msb_out16) -> dec_fir_async1/3(real1)
  bus_expand1/2(out15) -> dec_fir_async1/4(imag1)
  bus_expand1/3(out14) -> dec_fir_async1/5(real2)
  bus_expand1/4(out13) -> dec_fir_async1/6(imag2)
  bus_expand1/5(out12) -> dec_fir_async1/7(real3)
  bus_expand1/6(out11) -> dec_fir_async1/8(imag3)
  bus_expand1/7(out10) -> dec_fir_async1/9(real4)
  bus_expand1/8(out9) -> dec_fir_async1/10(imag4)
  bus_expand1/9(out8) -> dec_fir_async1/11(real5)
  bus_expand1/10(out7) -> dec_fir_async1/12(imag5)
  bus_expand1/11(out6) -> dec_fir_async1/13(real6)
  bus_expand1/12(out5) -> dec_fir_async1/14(imag6)
  bus_expand1/13(out4) -> dec_fir_async1/15(real7)
  bus_expand1/14(out3) -> dec_fir_async1/16(imag7)
  bus_expand1/15(out2) -> dec_fir_async1/17(real8)
  bus_expand1/16(lsb_out1) -> dec_fir_async1/18(imag8)
  bus_expand2/1(msb_out16) -> dec_fir_async1/19(real9)
  bus_expand2/2(out15) -> dec_fir_async1/20(imag9)
  bus_expand2/3(out14) -> dec_fir_async1/21(real10)
  bus_expand2/4(out13) -> dec_fir_async1/22(imag10)
  bus_expand2/5(out12) -> dec_fir_async1/23(real11)
  bus_expand2/6(out11) -> dec_fir_async1/24(imag11)
  bus_expand2/7(out10) -> dec_fir_async1/25(real12)
  bus_expand2/8(out9) -> dec_fir_async1/26(imag12)
  bus_expand2/9(out8) -> dec_fir_async1/27(real13)
  bus_expand2/10(out7) -> dec_fir_async1/28(imag13)
  bus_expand2/11(out6) -> dec_fir_async1/29(real14)
  bus_expand2/12(out5) -> dec_fir_async1/30(imag14)
  bus_expand2/13(out4) -> dec_fir_async1/31(real15)
  bus_expand2/14(out3) -> dec_fir_async1/32(imag15)
  bus_expand2/15(out2) -> dec_fir_async1/33(real16)
  bus_expand2/16(lsb_out1) -> dec_fir_async1/34(imag16)
  Delay5/1 -> bus_expand1/1(bus_in)
  bus_expand3/1(msb_out16) -> dec_fir_async1/35(real17)
  bus_expand3/2(out15) -> dec_fir_async1/36(imag17)
  bus_expand3/3(out14) -> dec_fir_async1/37(real18)
  bus_expand3/4(out13) -> dec_fir_async1/38(imag18)
  bus_expand3/5(out12) -> dec_fir_async1/39(real19)
  bus_expand3/6(out11) -> dec_fir_async1/40(imag19)
  bus_expand3/7(out10) -> dec_fir_async1/41(real20)
  bus_expand3/9(out8) -> dec_fir_async1/43(real21)
  bus_expand3/8(out9) -> dec_fir_async1/42(imag20)
  bus_expand3/10(out7) -> dec_fir_async1/44(imag21)
  bus_expand3/11(out6) -> dec_fir_async1/45(real22)
  bus_expand3/12(out5) -> dec_fir_async1/46(imag22)
  bus_expand3/13(out4) -> dec_fir_async1/47(real23)
  bus_expand3/14(out3) -> dec_fir_async1/48(imag23)
  bus_expand3/15(out2) -> dec_fir_async1/49(real24)
  bus_expand3/16(lsb_out1) -> dec_fir_async1/50(imag24)
  bus_expand4/1(msb_out16) -> dec_fir_async1/51(real25)
  bus_expand4/2(out15) -> dec_fir_async1/52(imag25)
  bus_expand4/3(out14) -> dec_fir_async1/53(real26)
  bus_expand4/4(out13) -> dec_fir_async1/54(imag26)
  bus_expand4/5(out12) -> dec_fir_async1/55(real27)
  bus_expand4/6(out11) -> dec_fir_async1/56(imag27)
  bus_expand4/7(out10) -> dec_fir_async1/57(real28)
  bus_expand4/8(out9) -> dec_fir_async1/58(imag28)
  bus_expand4/9(out8) -> dec_fir_async1/59(real29)
  bus_expand4/10(out7) -> dec_fir_async1/60(imag29)
  bus_expand4/11(out6) -> dec_fir_async1/61(real30)
  bus_expand4/13(out4) -> dec_fir_async1/63(real31)
  bus_expand4/12(out5) -> dec_fir_async1/62(imag30)
  bus_expand4/14(out3) -> dec_fir_async1/64(imag31)
  bus_expand4/15(out2) -> dec_fir_async1/65(real32)
  bus_expand4/16(lsb_out1) -> dec_fir_async1/66(imag32)
  Delay7/1 -> bus_expand3/1(bus_in)
  [mix_dvalid] -> Delay5/2, Delay8/2, Delay7/2
  Delay8/1 -> bus_expand2/1(bus_in)
  dec_fir_async1/2(dout) -> Delay10/1
  dec_fir_async1/3(dv_out) -> Delay9/1
  Delay9/1 -> [ddc_dvalid]
  Gateway Out4/1 -> To Workspace4/1
  bus_expand7/1(msb_out2) -> Gateway Out22/1
  bus_expand7/2(lsb_out1) -> Gateway Out23/1
  Gateway Out22/1 -> To Workspace22/1
  Gateway Out23/1 -> To Workspace5/1
  [mix_80_1] -> Register7/1
  [mix_80_0] -> Register4/1
  [mix_dvalid] -> Register5/3, Logical3/2, Register4/2, Register7/2
  Logical4/1 -> Delay12/1, Register6/2
  Register6/1 -> Logical4/1
  [mix_sync] -> Register6/1, Register6/3, Register5/2
  Assert1/1 -> Register5/1
  Inverter1/1 -> Assert1/1
  Register5/1 -> Delay13/1
  Delay13/1 -> Logical3/1, Inverter1/1
  Delay12/1 -> [dec_sync]
  Delay11/1 -> [dec_dv]
  Register4/1 -> [dec_d80_0]
  Register7/1 -> [dec_d80_1]
  Logical3/1 -> edge_detect2/1(in), Logical4/2
  edge_detect2/1(out) -> Delay11/1
  From16/1 -> bus_expand8/1(bus_in)
  Gateway Out10/1 -> To Workspace11/1
  bus_expand8/1(msb_out16) -> Gateway Out10/1
  Gateway Out12/1 -> To Workspace13/1
  bus_expand8/2(out15) -> Gateway Out12/1
  Gateway Out13/1 -> To Workspace14/1
  bus_expand8/3(out14) -> Gateway Out13/1
  Gateway Out14/1 -> To Workspace21/1
  bus_expand8/4(out13) -> Gateway Out14/1
  Gateway Out18/1 -> To Workspace24/1
  Gateway Out17/1 -> To Workspace16/1
  Gateway Out16/1 -> To Workspace23/1
  Gateway Out15/1 -> To Workspace15/1
  bus_expand8/5(out12) -> Gateway Out15/1
  bus_expand8/6(out11) -> Gateway Out16/1
  bus_expand8/7(out10) -> Gateway Out17/1
  bus_expand8/8(out9) -> Gateway Out18/1
  Gateway Out25/1 -> To Workspace19/1
  Gateway Out26/1 -> To Workspace27/1
  Gateway Out27/1 -> To Workspace20/1
  Gateway Out28/1 -> To Workspace28/1
  Gateway Out24/1 -> To Workspace26/1
  Gateway Out21/1 -> To Workspace18/1
  Gateway Out20/1 -> To Workspace25/1
  Gateway Out19/1 -> To Workspace17/1
  bus_expand8/9(out8) -> Gateway Out19/1
  bus_expand8/10(out7) -> Gateway Out20/1
  bus_expand8/11(out6) -> Gateway Out21/1
  bus_expand8/12(out5) -> Gateway Out24/1
  bus_expand8/13(out4) -> Gateway Out25/1
  bus_expand8/14(out3) -> Gateway Out26/1
  bus_expand8/15(out2) -> Gateway Out27/1
  bus_expand8/16(lsb_out1) -> Gateway Out28/1
  dec_fir_async1/1(sync_out) -> Gateway Out4/1, [ddc_sync]
  Delay10/1 -> bus_expand7/1(bus_in), [ddc_pol0]
  dec_fir_async2/1(sync_out) -> Terminator1/1
  dec_fir_async2/3(dv_out) -> Delay15/1
  dec_fir_async2/2(dout) -> Delay1/1
  Delay14/1 -> bus_expand6/1(bus_in)
  [mix_dvalid] -> Delay4/2, Delay14/2, Delay3/2
  Delay4/1 -> bus_expand9/1(bus_in)
  bus_expand10/16(lsb_out1) -> dec_fir_async2/66(imag32)
  bus_expand10/15(out2) -> dec_fir_async2/65(real32)
  bus_expand10/14(out3) -> dec_fir_async2/64(imag31)
  bus_expand10/12(out5) -> dec_fir_async2/62(imag30)
  bus_expand10/13(out4) -> dec_fir_async2/63(real31)
  bus_expand10/11(out6) -> dec_fir_async2/61(real30)
  bus_expand10/10(out7) -> dec_fir_async2/60(imag29)
  bus_expand10/9(out8) -> dec_fir_async2/59(real29)
  bus_expand10/8(out9) -> dec_fir_async2/58(imag28)
  bus_expand10/7(out10) -> dec_fir_async2/57(real28)
  bus_expand10/6(out11) -> dec_fir_async2/56(imag27)
  bus_expand10/5(out12) -> dec_fir_async2/55(real27)
  bus_expand10/4(out13) -> dec_fir_async2/54(imag26)
  bus_expand10/3(out14) -> dec_fir_async2/53(real26)
  bus_expand10/2(out15) -> dec_fir_async2/52(imag25)
  bus_expand10/1(msb_out16) -> dec_fir_async2/51(real25)
  bus_expand9/16(lsb_out1) -> dec_fir_async2/50(imag24)
  bus_expand9/15(out2) -> dec_fir_async2/49(real24)
  bus_expand9/14(out3) -> dec_fir_async2/48(imag23)
  bus_expand9/13(out4) -> dec_fir_async2/47(real23)
  bus_expand9/12(out5) -> dec_fir_async2/46(imag22)
  bus_expand9/11(out6) -> dec_fir_async2/45(real22)
  bus_expand9/10(out7) -> dec_fir_async2/44(imag21)
  bus_expand9/8(out9) -> dec_fir_async2/42(imag20)
  bus_expand9/9(out8) -> dec_fir_async2/43(real21)
  bus_expand9/7(out10) -> dec_fir_async2/41(real20)
  bus_expand9/6(out11) -> dec_fir_async2/40(imag19)
  bus_expand9/5(out12) -> dec_fir_async2/39(real19)
  bus_expand9/4(out13) -> dec_fir_async2/38(imag18)
  bus_expand9/3(out14) -> dec_fir_async2/37(real18)
  bus_expand9/2(out15) -> dec_fir_async2/36(imag17)
  bus_expand9/1(msb_out16) -> dec_fir_async2/35(real17)
  Delay3/1 -> bus_expand5/1(bus_in)
  bus_expand6/16(lsb_out1) -> dec_fir_async2/34(imag16)
  bus_expand6/15(out2) -> dec_fir_async2/33(real16)
  bus_expand6/14(out3) -> dec_fir_async2/32(imag15)
  bus_expand6/13(out4) -> dec_fir_async2/31(real15)
  bus_expand6/12(out5) -> dec_fir_async2/30(imag14)
  bus_expand6/11(out6) -> dec_fir_async2/29(real14)
  bus_expand6/10(out7) -> dec_fir_async2/28(imag13)
  bus_expand6/9(out8) -> dec_fir_async2/27(real13)
  bus_expand6/8(out9) -> dec_fir_async2/26(imag12)
  bus_expand6/7(out10) -> dec_fir_async2/25(real12)
  bus_expand6/6(out11) -> dec_fir_async2/24(imag11)
  bus_expand6/5(out12) -> dec_fir_async2/23(real11)
  bus_expand6/4(out13) -> dec_fir_async2/22(imag10)
  bus_expand6/3(out14) -> dec_fir_async2/21(real10)
  bus_expand6/2(out15) -> dec_fir_async2/20(imag9)
  bus_expand6/1(msb_out16) -> dec_fir_async2/19(real9)
  bus_expand5/16(lsb_out1) -> dec_fir_async2/18(imag8)
  bus_expand5/15(out2) -> dec_fir_async2/17(real8)
  bus_expand5/14(out3) -> dec_fir_async2/16(imag7)
  bus_expand5/13(out4) -> dec_fir_async2/15(real7)
  bus_expand5/12(out5) -> dec_fir_async2/14(imag6)
  bus_expand5/11(out6) -> dec_fir_async2/13(real6)
  bus_expand5/10(out7) -> dec_fir_async2/12(imag5)
  bus_expand5/9(out8) -> dec_fir_async2/11(real5)
  bus_expand5/8(out9) -> dec_fir_async2/10(imag4)
  bus_expand5/7(out10) -> dec_fir_async2/9(real4)
  bus_expand5/6(out11) -> dec_fir_async2/8(imag3)
  bus_expand5/5(out12) -> dec_fir_async2/7(real3)
  bus_expand5/4(out13) -> dec_fir_async2/6(imag2)
  bus_expand5/3(out14) -> dec_fir_async2/5(real2)
  bus_expand5/2(out15) -> dec_fir_async2/4(imag1)
  bus_expand5/1(msb_out16) -> dec_fir_async2/3(real1)
  [dec_sync] -> dec_fir_async2/1(sync_in)
  [dec_dv] -> dec_fir_async2/2(dv_in)
  [dec_d80_1] -> bus_expand10/1(bus_in), Delay4/1, Delay14/1, Delay3/1
  Delay1/1 -> [ddc_pol1]
  Delay15/1 -> Terminator/1
